simulink model "pidkgtt"  (R2020b)
settings: Solver=VariableStepAuto  StartTime=0.0  StopTime=10.0  RelTol=1e-3
libraries: pid_lib x3
settings Model: Creator=lamth  LastModifiedBy=lamth

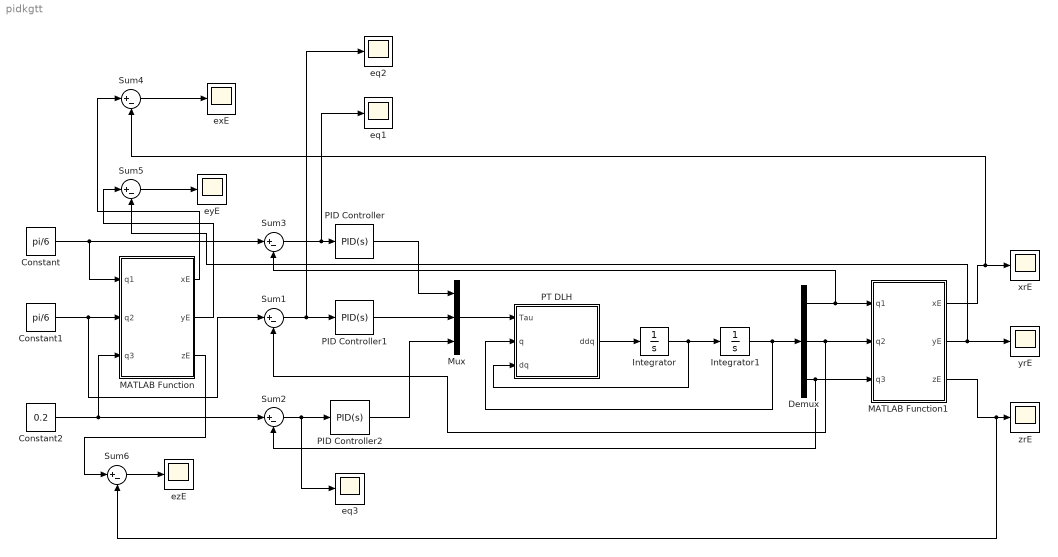
== system pidkgtt ==
  Constant : Constant  Value=pi/6
  Constant1 : Constant  Value=pi/6
  Constant2 : Constant  Value=0.2
  Demux : Demux  Outputs=3
  Integrator : Integrator
  Integrator1 : Integrator
  MATLAB Function : MATLAB Function  TreatAsAtomicUnit=on
  MATLAB Function1 : MATLAB Function  TreatAsAtomicUnit=on
  Mux : Mux  Inputs=3
  PID Controller : pid_lib/PID Controller  Controller=PID  Form=Parallel  TimeDomain=Continuous-time  UseExternalTs=off  SampleTime=-1  IntegratorMethod=Forward Euler  FilterMethod=Forward Euler  ControllerParametersSource=internal  P=7698.85885789315  I=36281.3363700772  D=178.250943289464  UseFilter=on  N=11649.8843622392  TunerSelectOption=Transfer Function Based (PID Tuner App)  InitialConditionSource=internal  InitialConditionForIntegrator=0  InitialConditionForFilter=0  DifferentiatorICPrevScaledInput=0  ExternalReset=none  TrackingMode=off  Kt=1  LimitOutput=off  SatLimitsSource=internal  UpperSaturationLimit=inf  LowerSaturationLimit=-inf  LinearizeAsGain=on  AntiWindupMode=none  Kb=1  POutMin=[]  POutMax=[]  IOutMin=[]  IOutMax=[]  DOutMin=[]  DOutMax=[]  NOutMin=[]  NOutMax=[]  SumOutMin=[]  SumOutMax=[]  SaturationOutMin=[]  SaturationOutMax=[]  PParamMin=[]  PParamMax=[]  IParamMin=[]  IParamMax=[]  DParamMin=[]  DParamMax=[]  NParamMin=[]  NParamMax=[]  KbParamMin=[]  KbParamMax=[]  KtParamMin=[]  KtParamMax=[]  KbOutMin=[]  KbOutMax=[]  KtOutMin=[]  KtOutMax=[]  IntegratorOutMin=[]  IntegratorOutMax=[]  FilterOutMin=[]  FilterOutMax=[]  SumI1OutMin=[]  SumI1OutMax=[]  SumI2OutMin=[]  SumI2OutMax=[]  SumI3OutMin=[]  SumI3OutMax=[]  SumI4OutMin=[]  SumI4OutMax=[]  SumDOutMin=[]  SumDOutMax=[]  DifferentiatorOutMin=[]  DifferentiatorOutMax=[]  FilterDiffOutCoefMin=[]  FilterDiffOutCoefMax=[]  ReciprocalOutMin=[]  ReciprocalOutMax=[]  SumDenOutMin=[]  SumDenOutMax=[]  SumNumOutMin=[]  SumNumOutMax=[]  DivideOutMin=[]  DivideOutMax=[]  UdiffTsProdOutMin=[]  UdiffTsProdOutMax=[]  NTsProdOutMin=[]  NTsProdOutMax=[]  UintegralTsProdOutMin=[]  UintegralTsProdOutMax=[]  UngainTsProdOutMin=[]  UngainTsProdOutMax=[]  IntegratorContinuousStateAttributes=''  IntegratorStateMustResolveToSignalObject=off  IntegratorRTWStateStorageClass=Auto  FilterContinuousStateAttributes=''  FilterStateMustResolveToSignalObject=off  FilterRTWStateStorageClass=Auto  ParallelPVariant=InternalParameters  IdealPVariant=Disabled  IVariant=InternalParameters  DVariant=InternalParameters  IntegratorVariant=Continuous  SatVariant=Disabled  AWVariant=Passthrough  PCopyVariant=Disabled  TRVariant=Disabled  FdbkBlocksVariant=Forward  IdealPFdbkVariant=Disabled  SatFdbkVariant=Disabled  DerivativeFilterVariant=ContFilter  NVariant=InternalParameters  NCopyVariant=Disabled  FilterICVariant=InternalICsFilter  IntegratorICVariant=InternalICs  ExternalResetVariant=Disabled  TRSumVariant=Passthrough  SumFdbkVariant=Disabled  SumVariant=Sum_PID  TsampFilterVariant=InternalTs  TsampNgainVariant=Passthrough  TsampIntegralVariant=Passthrough  ExternalSaturationOutDataTypeStr=Inherit: Same as second input
  PID Controller1 : pid_lib/PID Controller  Controller=PID  Form=Parallel  TimeDomain=Continuous-time  UseExternalTs=off  SampleTime=-1  IntegratorMethod=Forward Euler  FilterMethod=Forward Euler  ControllerParametersSource=internal  P=10259.2247290304  I=180710.920698239  D=80.0794481305014  UseFilter=on  N=25281.1710090221  TunerSelectOption=Transfer Function Based (PID Tuner App)  InitialConditionSource=internal  InitialConditionForIntegrator=0  InitialConditionForFilter=0  DifferentiatorICPrevScaledInput=0  ExternalReset=none  TrackingMode=off  Kt=1  LimitOutput=off  SatLimitsSource=internal  UpperSaturationLimit=inf  LowerSaturationLimit=-inf  LinearizeAsGain=on  AntiWindupMode=none  Kb=1  POutMin=[]  POutMax=[]  IOutMin=[]  IOutMax=[]  DOutMin=[]  DOutMax=[]  NOutMin=[]  NOutMax=[]  SumOutMin=[]  SumOutMax=[]  SaturationOutMin=[]  SaturationOutMax=[]  PParamMin=[]  PParamMax=[]  IParamMin=[]  IParamMax=[]  DParamMin=[]  DParamMax=[]  NParamMin=[]  NParamMax=[]  KbParamMin=[]  KbParamMax=[]  KtParamMin=[]  KtParamMax=[]  KbOutMin=[]  KbOutMax=[]  KtOutMin=[]  KtOutMax=[]  IntegratorOutMin=[]  IntegratorOutMax=[]  FilterOutMin=[]  FilterOutMax=[]  SumI1OutMin=[]  SumI1OutMax=[]  SumI2OutMin=[]  SumI2OutMax=[]  SumI3OutMin=[]  SumI3OutMax=[]  SumI4OutMin=[]  SumI4OutMax=[]  SumDOutMin=[]  SumDOutMax=[]  DifferentiatorOutMin=[]  DifferentiatorOutMax=[]  FilterDiffOutCoefMin=[]  FilterDiffOutCoefMax=[]  ReciprocalOutMin=[]  ReciprocalOutMax=[]  SumDenOutMin=[]  SumDenOutMax=[]  SumNumOutMin=[]  SumNumOutMax=[]  DivideOutMin=[]  DivideOutMax=[]  UdiffTsProdOutMin=[]  UdiffTsProdOutMax=[]  NTsProdOutMin=[]  NTsProdOutMax=[]  UintegralTsProdOutMin=[]  UintegralTsProdOutMax=[]  UngainTsProdOutMin=[]  UngainTsProdOutMax=[]  IntegratorContinuousStateAttributes=''  IntegratorStateMustResolveToSignalObject=off  IntegratorRTWStateStorageClass=Auto  FilterContinuousStateAttributes=''  FilterStateMustResolveToSignalObject=off  FilterRTWStateStorageClass=Auto  ParallelPVariant=InternalParameters  IdealPVariant=Disabled  IVariant=InternalParameters  DVariant=InternalParameters  IntegratorVariant=Continuous  SatVariant=Disabled  AWVariant=Passthrough  PCopyVariant=Disabled  TRVariant=Disabled  FdbkBlocksVariant=Forward  IdealPFdbkVariant=Disabled  SatFdbkVariant=Disabled  DerivativeFilterVariant=ContFilter  NVariant=InternalParameters  NCopyVariant=Disabled  FilterICVariant=InternalICsFilter  IntegratorICVariant=InternalICs  ExternalResetVariant=Disabled  TRSumVariant=Passthrough  SumFdbkVariant=Disabled  SumVariant=Sum_PID  TsampFilterVariant=InternalTs  TsampNgainVariant=Passthrough  TsampIntegralVariant=Passthrough  ExternalSaturationOutDataTypeStr=Inherit: Same as second input
  PID Controller2 : pid_lib/PID Controller  Controller=PID  Form=Parallel  TimeDomain=Continuous-time  UseExternalTs=off  SampleTime=-1  IntegratorMethod=Forward Euler  FilterMethod=Forward Euler  ControllerParametersSource=internal  P=50  I=30  D=20  UseFilter=on  N=100  TunerSelectOption=Transfer Function Based (PID Tuner App)  InitialConditionSource=internal  InitialConditionForIntegrator=0  InitialConditionForFilter=0  DifferentiatorICPrevScaledInput=0  ExternalReset=none  TrackingMode=off  Kt=1  LimitOutput=off  SatLimitsSource=internal  UpperSaturationLimit=inf  LowerSaturationLimit=-inf  LinearizeAsGain=on  AntiWindupMode=none  Kb=1  POutMin=[]  POutMax=[]  IOutMin=[]  IOutMax=[]  DOutMin=[]  DOutMax=[]  NOutMin=[]  NOutMax=[]  SumOutMin=[]  SumOutMax=[]  SaturationOutMin=[]  SaturationOutMax=[]  PParamMin=[]  PParamMax=[]  IParamMin=[]  IParamMax=[]  DParamMin=[]  DParamMax=[]  NParamMin=[]  NParamMax=[]  KbParamMin=[]  KbParamMax=[]  KtParamMin=[]  KtParamMax=[]  KbOutMin=[]  KbOutMax=[]  KtOutMin=[]  KtOutMax=[]  IntegratorOutMin=[]  IntegratorOutMax=[]  FilterOutMin=[]  FilterOutMax=[]  SumI1OutMin=[]  SumI1OutMax=[]  SumI2OutMin=[]  SumI2OutMax=[]  SumI3OutMin=[]  SumI3OutMax=[]  SumI4OutMin=[]  SumI4OutMax=[]  SumDOutMin=[]  SumDOutMax=[]  DifferentiatorOutMin=[]  DifferentiatorOutMax=[]  FilterDiffOutCoefMin=[]  FilterDiffOutCoefMax=[]  ReciprocalOutMin=[]  ReciprocalOutMax=[]  SumDenOutMin=[]  SumDenOutMax=[]  SumNumOutMin=[]  SumNumOutMax=[]  DivideOutMin=[]  DivideOutMax=[]  UdiffTsProdOutMin=[]  UdiffTsProdOutMax=[]  NTsProdOutMin=[]  NTsProdOutMax=[]  UintegralTsProdOutMin=[]  UintegralTsProdOutMax=[]  UngainTsProdOutMin=[]  UngainTsProdOutMax=[]  IntegratorContinuousStateAttributes=''  IntegratorStateMustResolveToSignalObject=off  IntegratorRTWStateStorageClass=Auto  FilterContinuousStateAttributes=''  FilterStateMustResolveToSignalObject=off  FilterRTWStateStorageClass=Auto  ParallelPVariant=InternalParameters  IdealPVariant=Disabled  IVariant=InternalParameters  DVariant=InternalParameters  IntegratorVariant=Continuous  SatVariant=Disabled  AWVariant=Passthrough  PCopyVariant=Disabled  TRVariant=Disabled  FdbkBlocksVariant=Forward  IdealPFdbkVariant=Disabled  SatFdbkVariant=Disabled  DerivativeFilterVariant=ContFilter  NVariant=InternalParameters  NCopyVariant=Disabled  FilterICVariant=InternalICsFilter  IntegratorICVariant=InternalICs  ExternalResetVariant=Disabled  TRSumVariant=Passthrough  SumFdbkVariant=Disabled  SumVariant=Sum_PID  TsampFilterVariant=InternalTs  TsampNgainVariant=Passthrough  TsampIntegralVariant=Passthrough  ExternalSaturationOutDataTypeStr=Inherit: Same as second input
  PT DLH : MATLAB Function  TreatAsAtomicUnit=on
  Sum{1..6} (6 alike) : Sum  Inputs=|+-
  eq1 : Scope
  eq2 : Scope
  eq3 : Scope
  exE : Scope
  eyE : Scope
  ezE : Scope
  xrE : Scope
  yrE : Scope
  zrE : Scope
  wires:
  PT DLH/1(ddq) -> Integrator/1
  PID Controller1/1 -> Mux/2
  PID Controller/1 -> Mux/1
  Integrator/1 -> Integrator1/1, PT DLH/3(dq)
  Integrator1/1 -> Demux/1, PT DLH/2(q)
  PID Controller2/1 -> Mux/3
  Sum3/1 -> eq1/1, PID Controller/1
  Mux/1 -> PT DLH/1(Tau)
  Sum2/1 -> eq3/1, PID Controller2/1
  Sum1/1 -> eq2/1, PID Controller1/1
  Demux/2 -> Sum1/2, MATLAB Function1/2(q2)
  Demux/3 -> MATLAB Function1/3(q3), Sum2/2
  Demux/1 -> Sum3/2, MATLAB Function1/1(q1)
  Sum4/1 -> exE/1
  Sum5/1 -> eyE/1
  Sum6/1 -> ezE/1
  MATLAB Function1/2(yE) -> Sum5/2, yrE/1
  MATLAB Function1/3(zE) -> Sum6/2, zrE/1
  MATLAB Function1/1(xE) -> xrE/1, Sum4/2
  Constant/1 -> MATLAB Function/1(q1), Sum3/1
  Constant2/1 -> MATLAB Function/3(q3), Sum2/1
  Constant1/1 -> MATLAB Function/2(q2), Sum1/1
  MATLAB Function/3(zE) -> Sum6/1
  MATLAB Function/2(yE) -> Sum5/1
  MATLAB Function/1(xE) -> Sum4/1

== matlab function pidkgtt/PT DLH ==
  data: Tau input; q input; ddq output; dq input
function ddq  = fcn(Tau,q,dq)
[m1,m2,m3,L1,L2,L3,I1x,I1y,I1z,I2x,I2y,I2z,I3x,I3y,I3z]=parameter ();

q=zeros(3,1);
dq=zeros(3,1);

% Khai bao ma tran khoi luong M
M=zeros(3,3);
M(1,1)= (9/4)*m1*L1^2+I1z+3*m2*L2*L1*cos(q(2))+L1^2*m2+(9/4)*m2*L2^2+I2y+2*m3*L2*L1*cos(q(2))+3*m3*L1*q(3)*sin(q(2))+L1^2*m3+L2^2*m3+(9/4)*m3*q(3)^2+I3y;
M(1,2)= (3/2)*m2*L2*L1*cos(q(2))+(9/4)*m2*L2^2+I2y+m3*L2*L1*cos(q(2))+(3/2)*m3*L1*q(3)*sin(q(2))+L2^2*m3+(9/4)*m3*q(3)^2+I3y;
M(1,3)= -(3/2)*L1*m3*cos(q(2))-(3/2)*L2*m3;


M(2,1)=(3/2)*m2*L2*L1*cos(q(2))+(9/4)*m2*L2^2+I2y+m3*L2*L1*cos(q(2))+(3/2)*m3*L1*q(3)*sin(q(2))+L2^2*m3+(9/4)*m3*q(3)^2+I3y;
M(2,2)=(9/4)*m2*L2^2+I2y+L2^2*m3+(9/4)*m3*q(3)^2+I3y;
M(2,3)=-(3/2)*L2*m3;

M(3,1)=-(3/2)*L1*m3*cos(q(2))-(3/2)*L2*m3;
M(3,2)=-(3/2)*L2*m3;
M(3,3)=(9/4)*m3;

% Khai bao ma tran Coriolis C
%h=-m2*L1*Lc2*sin(q(2));
Co=zeros(3,3);
Co(1,1)=-3*L1*L2*sin(q(2))*dq(2)*m2-2*L1*L2*sin(q(2))*dq(2)*m3+3*L1*cos(q(2))*dq(2)*m3*q(3)+3*L1*m3*sin(q(2))*dq(3)+(9/2)*m3*q(3)*dq(3);
Co(1,2)=-(3/2)*L1*L2*sin(q(2))*dq(2)*m2-L1*L2*sin(q(2))*dq(2)*m3+(3/2)*L1*cos(q(2))*dq(2)*m3*q(3)+(3/2)*L1*m3*sin(q(2))*dq(3)+(9/2)*m3*q(3)*dq(3);
Co(1,3)=(3/2)*L1*m3*sin(q(2))*dq(2);


Co(2,1)=(3/2)*L1*L2*sin(q(2))*dq(1)*m2+L1*L2*sin(q(2))*dq(1)*m3-(3/4)*L1*L2*sin(q(2))*dq(2)*m2-(1/2)*L1*L2*sin(q(2))*dq(2)*m3-(3/2)*L1*cos(q(2))*dq(1)*m3*q(3)+(3/4)*L1*cos(q(2))*dq(2)*m3*q(3)+(3/4)*L1*m3*sin(q(2))*dq(3)+(9/2)*m3*q(3)*dq(3);
Co(2,2)=(3/4)*L1*L2*sin(q(2))*dq(1)*m2+(1/2)*L1*L2*sin(q(2))*dq(1)*m3-(3/4)*L1*cos(q(2))*dq(1)*m3*q(3)+(9/2)*m3*q(3)*dq(3);
Co(2,3)=-(3/4)*L1*m3*sin(q(2))*dq(1);


Co(3,1)=-(3/2)*L1*m3*sin(q(2))*dq(1)+(3/4)*L1*m3*sin(q(2))*dq(2)-(9/4)*dq(1)*m3*q(3)-(9/4)*m3*q(3)*dq(2);
Co(3,2)=-(3/4)*L1*m3*sin(q(2))*dq(1)-(9/4)*dq(1)*m3*q(3)-(9/4)*m3*q(3)*dq(2);
Co(3,3)=0;

% Ma tran the nang hap dan
G=zeros(3,1);
G(1,1)=15*m1*L1*cos(q(1))+10*m2*L1*cos(q(1))+10*m3*L1*cos(q(1))+15*m2*L2*cos(q(1)+q(2))+10*m3*L2*cos(q(1)+q(2))+15*m3*sin(q(1)+q(2))*q(3);
G(2,1)=15*m2*L2*cos(q(1)+q(2))+10*m3*L2*cos(q(1)+q(2))+15*m3*sin(q(1)+q(2))*q(3);
G(3,1)=-15*m3*cos(q(1)+q(2));


% Pt DLH
ddq=inv(M)*(Tau-Co*dq-G);

== matlab function pidkgtt/MATLAB Function ==
  data: q1 input; xE output; q2 input; q3 input; yE output; zE output
function [xE,yE,zE] = DHT(q1,q2,q3)

[m1,m2,m3,L1,L2,L3,I1x,I1y,I1z,I2x,I2y,I2z,I3x,I3y,I3z]=parameter ();

xE=sin(q1 + q2) * q3 + L2 * cos(q1 + q2) + L1 * cos(q1);
yE=-cos(q1 + q2) * q3 + L2 * sin(q1 + q2) + L1 * sin(q1);
zE=0;

== matlab function pidkgtt/MATLAB Function1 ==
  data: q1 input; xE output; q2 input; q3 input; yE output; zE output
function [xE,yE,zE] = DHT(q1,q2,q3)
[m1,m2,m3,L1,L2,L3,I1x,I1y,I1z,I2x,I2y,I2z,I3x,I3y,I3z]=parameter ();

xE=sin(q1 + q2) * q3 + L2 * cos(q1 + q2) + L1 * cos(q1);
yE=-cos(q1 + q2) * q3 + L2 * sin(q1 + q2) + L1 * sin(q1);
zE=0;
